simulink model "MSD_sim"  (R2021a)
settings: Solver=FixedStepAuto  StartTime=0.0  StopTime=inf  FixedStep=0.01  RelTol=1e-3
undefined symbols (not defined in the file): b, denC, k, m, numC
settings Model: EnablePacing=on  Creator=vcichella  LastModifiedBy=vcichella

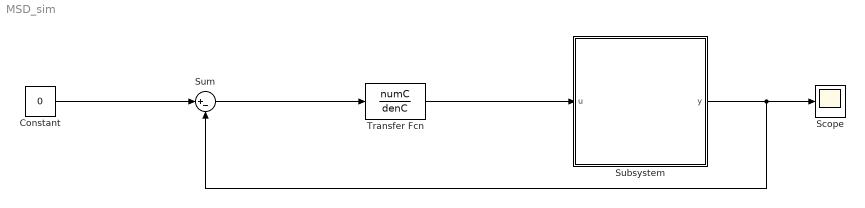
== system MSD_sim ==
  Constant : Constant  Value=0
  Scope : Scope
  Subsystem : Subsystem
  Sum : Sum  Inputs=|+-
  Transfer Fcn : TransferFcn  Numerator=numC  Denominator=denC
  wires:
  Subsystem/1(y) -> Sum/2, Scope/1
  Sum/1 -> Transfer Fcn/1
  Transfer Fcn/1 -> Subsystem/1(u)
  Constant/1 -> Sum/1

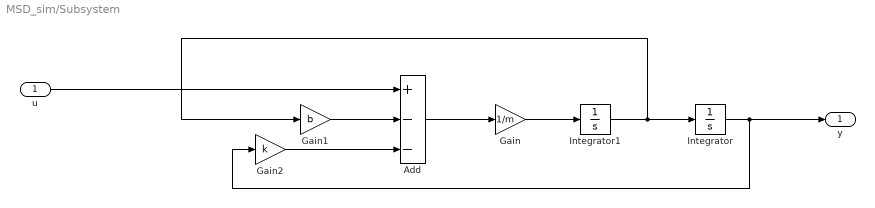
== system MSD_sim/Subsystem ==
  u : Inport
  Add : Sum  Inputs=+--
  Gain : Gain  Gain=1/m
  Gain1 : Gain  Gain=b
  Gain2 : Gain  Gain=k
  Integrator : Integrator
  Integrator1 : Integrator
  y : Outport
  wires:
  Integrator/1 -> y/1, Gain2/1
  Gain2/1 -> Add/3
  Add/1 -> Gain/1
  Integrator1/1 -> Gain1/1, Integrator/1
  Gain/1 -> Integrator1/1
  Gain1/1 -> Add/2
  u/1 -> Add/1
